simulink model "verify_Shading_Control_mdl"  (R2016b)
settings: Solver=ode45  StartTime=0.0  StopTime=3*24*3600  MaxStep=300  RelTol=1e-3  EnableMultiTasking=on
libraries: simulink x2, carnot x2
settings Model: Creator=drhf  LastModifiedBy=drhf
settings DataIOCC: SaveFormat=Array  SignalLoggingSaveFormat=ModelDataLogs
settings OptimizationCC: ExpressionDepthLimit=2147483647  LifeSpan=inf
settings DebuggingCC: UnderspecifiedInitializationDetection=Classic  MergeDetectMultiDrivingBlocksExec=none  SolverPrmCheckMsg=warning  FcnCallInpInsideContextMsg=warning  StateNameClashWarn=warning  SFUnexpectedBacktrackingDiag=warning  SFNoUnconditionalDefaultTransitionDiag=warning  SFExecutionAtInitializationDiag=none
settings HardwareCC: ProdBitPerPointer=32  ProdBitPerSizeT=32  ProdBitPerPtrDiffT=32  ProdLargestAtomicFloat=None  ProdIntDivRoundTo=Undefined  ProdEndianess=Unspecified  ProdWordSize=32  ProdHWDeviceType=32-bit Generic
settings ModelReferenceCC: PropagateSignalLabelsOutOfModel=off
settings GRTTargetCC: TargetLangStandard=C89/C90 (ANSI)  GeneratePreprocessorConditionals=Disable all  CombineOutputUpdateFcns=off  GRTInterface=on
settings ConfigComp: CovMetricSettings=dw  CovHtmlReporting=on  CovSaveCumulativeToWorkspaceVar=on  CovSaveSingleToWorkspaceVar=on  CovExternalEMLEnable=off

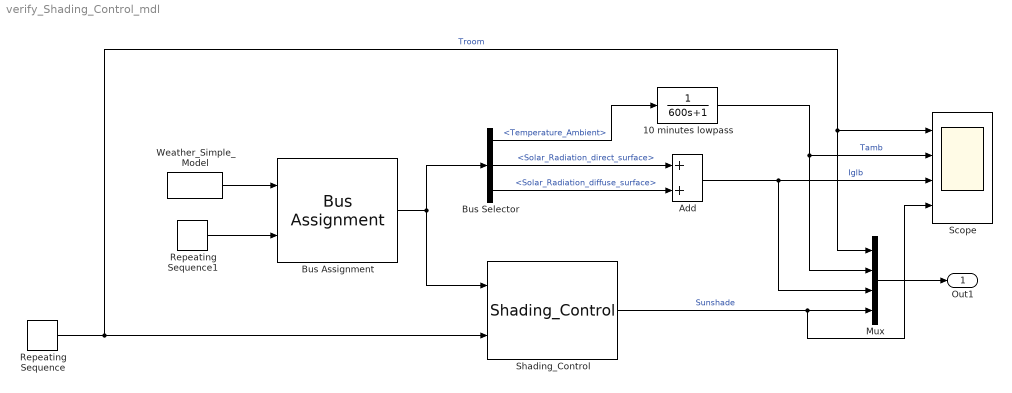
== system verify_Shading_Control_mdl ==
  10 minutes lowpass : TransferFcn  Denominator=[600 1]
  Add : Sum
  Bus Assignment : BusAssignment  AssignedSignals=Temperature_Ambient
  Bus Selector : BusSelector  OutputSignals=Temperature_Ambient,Solar_Radiation_direct_surface,Solar_Radiation_diffuse_surface
  Mux : Mux
  Repeating Sequence : simulink/Sources/Repeating Sequence  rep_seq_t="[0  24 24.1 34 34.1 38 38.1 48 48.1 72]*3600"  rep_seq_y="[25 25 20   20  25  25  20   20  25   25]"
  Repeating Sequence1 : simulink/Sources/Repeating Sequence  rep_seq_t="[0  58 58.1 62 62.1 72]*3600"  rep_seq_y="[20 20  0    0  20    20]"
  Scope : Scope  NumInputPorts=4
  Shading_Control : carnot/Control/Shading_Control  TroomShadeOn=23.8  TroomShadeOff=22.8  SolarShadeOn=300  SolarShadeOff=200  max_shade=0.95
  Weather_Simple_Model : carnot/Weather/Weather_Simple_Model  lat=-20  Ibn=900  Idg=100  tamb=5  deltaTsky=-6  rh=50  precip="10e-3/24/3600           % 10 mm in 24 h"  cloud=0.125  p=1013e2  vw=1  wdir=270
  Out1 : Outport
  wires:
  Shading_Control/1 -> Scope/4, Mux/4  "Sunshade"
  Repeating Sequence/1 -> Shading_Control/2, Scope/1, Mux/1  "Troom"
  Bus Assignment/1 -> Shading_Control/1, Bus Selector/1
  Mux/1 -> Out1/1
  Bus Selector/1 -> 10 minutes lowpass/1  "<Temperature_Ambient>"
  Bus Selector/2 -> Add/1  "<Solar_Radiation_direct_surface>"
  Bus Selector/3 -> Add/2  "<Solar_Radiation_diffuse_surface>"
  Add/1 -> Scope/3, Mux/3  "Iglb"
  Weather_Simple_Model/1 -> Bus Assignment/1
  Repeating Sequence1/1 -> Bus Assignment/2
  10 minutes lowpass/1 -> Mux/2, Scope/2  "Tamb"
